simulink model "Forward_and_inverse_Both"  (R2024b)
settings: Solver=VariableStepAuto  StartTime=0.0  StopTime=7  MaxStep=0.005  RelTol=1e-3
model workspace: external: MATLAB File D:\OneDrive - itc.edu.kh\V4_robot_arm\Import_arm6\Test_Assembly_DataFile.m (data not in the file)
values from neighbouring files (symbols this model uses):
  Reach_max = max(REACH_MAX)    [Workspace_sample.m]
  Reach_min = max(REACH_MIN)    [Workspace_sample.m]
undefined symbols (not defined in the file or in its folder): DiscIntNeverNeededParam, initialPose, maxAngularAcc, maxAngularVel, maxLinearAcc, maxLinearVel, poseTol, smiData, Ts, wps1, X, Y, Z
libraries: sm_lib x140, nesl_utility x52, stmnucleolib x12, simulink x4, vrlib x2, vexcommonlib x2, robotcorelib x2
(part 5 of 6)

== system Forward_and_inverse_Both/Simscape Robot2/Link4_v2_1_RIGID1 ==
  ReferenceFrame : sm_lib/Frames and Transforms/Reference Frame
  Solid : sm_lib/Body Elements/File Solid  ExtGeomFileName=D:\Test_hardware\simscape\Solidworks FIle\Link4_v2_Default_sldprt.STEP  UnitType=FromFile  ExtGeomFileUnits=m  StepReaderType=HEX  ExportConvexHullGeometry=off  InertiaType=Custom  BasedOnType=DensityFromFile  Density=1000  DensityUnits=kg/m^3  Mass=smiData.Solid(7).mass  MassUnits=kg  CenterOfMass=smiData.Solid(7).CoM  CenterOfMassUnits=mm  MomentsOfInertia=smiData.Solid(7).MoI  MomentsOfInertiaUnits=kg*mm^2  ProductsOfInertia=smiData.Solid(7).PoI  ProductsOfInertiaUnits=kg*mm^2  GraphicType=FromGeometry  MarkerShape=Sphere  MarkerSize=10  GraphicVisPropType=SimpleVisualProperties  GraphicDiffuseColor=[0.0 1.0 1.0]  GraphicOpacity=smiData.Solid(7).opacity  GraphicSpecularColor=[0.1 0.1 0.1 1.0]  GraphicAmbientColor=[0.15 0.15 0.15 1.0]  GraphicEmissiveColor=[0.5 0.5 0.5 1.0]  GraphicShininess=75  DoExposeReferenceFrame=on  SerializedFrames=<Frames/>
  Transform : sm_lib/Frames and Transforms/Rigid Transform  RotationMethod=ArbitraryAxis  FollAlignAxisA=+X  BaseAlignAxisA=+Y  FollAlignAxisB=+Y  BaseAlignAxisB=+Z  RotationStandardAxis=+Z  RotationAngle=smiData.RigidTransform(2).angle  RotationAngleUnits=rad  RotationArbitraryAxis=smiData.RigidTransform(2).axis  RotationSequenceAxes=FollowerAxes  RotationSequence=XYX  RotationSequenceAngles=[0 0 0]  RotationSequenceAnglesUnits=deg  RotationMatrix=[1 0 0; 0 1 0; 0 0 1]  Quaternion=[1 0 0 0]  TranslationMethod=Cartesian  TranslationCartesianOffset=smiData.RigidTransform(2).translation  TranslationCartesianOffsetUnits=mm  TranslationStandardAxis=+Z  TranslationStandardOffset=0  TranslationStandardOffsetUnits=mm  TranslationROffset=0  TranslationROffsetUnits=m  TranslationThetaOffset=0  TranslationThetaOffsetUnits=deg  TranslationZOffset=0  TranslationZOffsetUnits=m
  Transform1 : sm_lib/Frames and Transforms/Rigid Transform  RotationMethod=ArbitraryAxis  FollAlignAxisA=+X  BaseAlignAxisA=+Y  FollAlignAxisB=+Y  BaseAlignAxisB=+Z  RotationStandardAxis=+Z  RotationAngle=smiData.RigidTransform(3).angle  RotationAngleUnits=rad  RotationArbitraryAxis=smiData.RigidTransform(3).axis  RotationSequenceAxes=FollowerAxes  RotationSequence=XYX  RotationSequenceAngles=[0 0 0]  RotationSequenceAnglesUnits=deg  RotationMatrix=[1 0 0; 0 1 0; 0 0 1]  Quaternion=[1 0 0 0]  TranslationMethod=Cartesian  TranslationCartesianOffset=smiData.RigidTransform(3).translation  TranslationCartesianOffsetUnits=mm  TranslationStandardAxis=+Z  TranslationStandardOffset=0  TranslationStandardOffsetUnits=mm  TranslationROffset=0  TranslationROffsetUnits=m  TranslationThetaOffset=0  TranslationThetaOffsetUnits=deg  TranslationZOffset=0  TranslationZOffsetUnits=m
  F : PMIOPort  Side=Left
  F1 : PMIOPort  Port=2  Side=Right
  connections:
  ReferenceFrame/RConn1 -- Transform/LConn1 -- Transform1/LConn1 -- Solid/RConn1
  Transform/RConn1 -- F/RConn1
  Transform1/RConn1 -- F1/RConn1

== system Forward_and_inverse_Both/Simscape Robot2/Link5_v2_1_RIGID1 ==
  ReferenceFrame : sm_lib/Frames and Transforms/Reference Frame
  Solid : sm_lib/Body Elements/File Solid  ExtGeomFileName=D:\Test_hardware\simscape\Solidworks FIle\Link5_v2_Default_sldprt.STEP  UnitType=FromFile  ExtGeomFileUnits=m  StepReaderType=HEX  ExportConvexHullGeometry=off  InertiaType=Custom  BasedOnType=DensityFromFile  Density=1000  DensityUnits=kg/m^3  Mass=smiData.Solid(1).mass  MassUnits=kg  CenterOfMass=smiData.Solid(1).CoM  CenterOfMassUnits=mm  MomentsOfInertia=smiData.Solid(1).MoI  MomentsOfInertiaUnits=kg*mm^2  ProductsOfInertia=smiData.Solid(1).PoI  ProductsOfInertiaUnits=kg*mm^2  GraphicType=FromGeometry  MarkerShape=Sphere  MarkerSize=10  GraphicVisPropType=SimpleVisualProperties  GraphicDiffuseColor=[0.2 1.0 1.0]  GraphicOpacity=smiData.Solid(1).opacity  GraphicSpecularColor=[0.5 0.5 0.5 1.0]  GraphicAmbientColor=[0.15 0.15 0.15 1.0]  GraphicEmissiveColor=[0.0 0.0 0.0 1.0]  GraphicShininess=75  DoExposeReferenceFrame=on  SerializedFrames=<Frames/>
  Transform : sm_lib/Frames and Transforms/Rigid Transform  RotationMethod=ArbitraryAxis  FollAlignAxisA=+X  BaseAlignAxisA=+Y  FollAlignAxisB=+Y  BaseAlignAxisB=+Z  RotationStandardAxis=+Z  RotationAngle=smiData.RigidTransform(4).angle  RotationAngleUnits=rad  RotationArbitraryAxis=smiData.RigidTransform(4).axis  RotationSequenceAxes=FollowerAxes  RotationSequence=XYX  RotationSequenceAngles=[0 0 0]  RotationSequenceAnglesUnits=deg  RotationMatrix=[1 0 0; 0 1 0; 0 0 1]  Quaternion=[1 0 0 0]  TranslationMethod=Cartesian  TranslationCartesianOffset=smiData.RigidTransform(4).translation  TranslationCartesianOffsetUnits=mm  TranslationStandardAxis=+Z  TranslationStandardOffset=0  TranslationStandardOffsetUnits=mm  TranslationROffset=0  TranslationROffsetUnits=m  TranslationThetaOffset=0  TranslationThetaOffsetUnits=deg  TranslationZOffset=0  TranslationZOffsetUnits=m
  Transform1 : sm_lib/Frames and Transforms/Rigid Transform  RotationMethod=ArbitraryAxis  FollAlignAxisA=+X  BaseAlignAxisA=+Y  FollAlignAxisB=+Y  BaseAlignAxisB=+Z  RotationStandardAxis=+Z  RotationAngle=smiData.RigidTransform(9).angle  RotationAngleUnits=rad  RotationArbitraryAxis=smiData.RigidTransform(9).axis  RotationSequenceAxes=FollowerAxes  RotationSequence=XYX  RotationSequenceAngles=[0 0 0]  RotationSequenceAnglesUnits=deg  RotationMatrix=[1 0 0; 0 1 0; 0 0 1]  Quaternion=[1 0 0 0]  TranslationMethod=Cartesian  TranslationCartesianOffset=smiData.RigidTransform(9).translation  TranslationCartesianOffsetUnits=mm  TranslationStandardAxis=+Z  TranslationStandardOffset=0  TranslationStandardOffsetUnits=mm  TranslationROffset=0  TranslationROffsetUnits=m  TranslationThetaOffset=0  TranslationThetaOffsetUnits=deg  TranslationZOffset=0  TranslationZOffsetUnits=m
  F : PMIOPort  Side=Left
  F1 : PMIOPort  Port=2  Side=Right
  connections:
  ReferenceFrame/RConn1 -- Transform/LConn1 -- Transform1/LConn1 -- Solid/RConn1
  Transform/RConn1 -- F/RConn1
  Transform1/RConn1 -- F1/RConn1

== system Forward_and_inverse_Both/Subsystem/Joint 1 R1 = counter-clockwise L1 = clockwise ==
  L1 : Inport
  R1 : Inport  Port=2
  delta : Inport  Port=3
  pos_prev : Inport  Port=4
  MATLAB Function1 : MATLAB Function  TreatAsAtomicUnit=on
  Position limiter : MATLAB Function  TreatAsAtomicUnit=on
  Joint_1 : Outport
  wires:
  R1/1 -> MATLAB Function1/2(buttonR)
  Position limiter/1(y) -> Joint_1/1
  MATLAB Function1/1(pos) -> Position limiter/1(pos)
  L1/1 -> MATLAB Function1/1(buttonL)
  delta/1 -> Position limiter/2(delta), MATLAB Function1/4(delta)
  pos_prev/1 -> MATLAB Function1/3(pos_prev)

== system Forward_and_inverse_Both/Subsystem/Joint 6 L = counter-clockwise R = clockwise ==
  Dpad L : Inport
  Dpad R : Inport  Port=2
  delta : Inport  Port=3
  pos_prev : Inport  Port=4
  MATLAB Function1 : MATLAB Function  TreatAsAtomicUnit=on
  Position limiter : MATLAB Function  TreatAsAtomicUnit=on
  Joint_6 : Outport
  wires:
  delta/1 -> MATLAB Function1/4(delta), Position limiter/2(delta)
  Dpad L/1 -> MATLAB Function1/1(buttonL)
  MATLAB Function1/1(pos) -> Position limiter/1(pos)
  Position limiter/1(y) -> Joint_6/1
  Dpad R/1 -> MATLAB Function1/2(buttonR)
  pos_prev/1 -> MATLAB Function1/3(pos_prev)

== system Forward_and_inverse_Both/Subsystem20/Joint 1 R1 = counter-clockwise L1 = clockwise ==
  L1 : Inport
  R1 : Inport  Port=2
  delta : Inport  Port=3
  pos_prev : Inport  Port=4
  MATLAB Function1 : MATLAB Function  TreatAsAtomicUnit=on
  Position limiter : MATLAB Function  TreatAsAtomicUnit=on
  Joint_1 : Outport
  wires:
  R1/1 -> MATLAB Function1/2(buttonR)
  Position limiter/1(y) -> Joint_1/1
  MATLAB Function1/1(pos) -> Position limiter/1(pos)
  L1/1 -> MATLAB Function1/1(buttonL)
  delta/1 -> Position limiter/2(delta), MATLAB Function1/4(delta)
  pos_prev/1 -> MATLAB Function1/3(pos_prev)

== system Forward_and_inverse_Both/Subsystem20/Joint 6 L = counter-clockwise R = clockwise ==
  Dpad L : Inport
  Dpad R : Inport  Port=2
  delta : Inport  Port=3
  pos_prev : Inport  Port=4
  MATLAB Function1 : MATLAB Function  TreatAsAtomicUnit=on
  Position limiter : MATLAB Function  TreatAsAtomicUnit=on
  Joint_6 : Outport
  wires:
  delta/1 -> MATLAB Function1/4(delta), Position limiter/2(delta)
  Dpad L/1 -> MATLAB Function1/1(buttonL)
  MATLAB Function1/1(pos) -> Position limiter/1(pos)
  Position limiter/1(y) -> Joint_6/1
  Dpad R/1 -> MATLAB Function1/2(buttonR)
  pos_prev/1 -> MATLAB Function1/3(pos_prev)

== matlab function Forward_and_inverse_Both/Forward_Kinematic_Good4 ==
  data: Px output; Py output; Pz output; th1 input; th2 input; th3 input; th4 input; th5 input; th6 input
function [Px,Py,Pz] = forward_kinematics(th1, th2, th3, th4, th5, th6)
%All length in mm
l1=276;
l2=306;
a=79.75;
l3=160;
l4=227;
l5=70;
l6=38;
    % Compute DH transformation matrices
    A0 = dh_matrix(0    , 0     ,l1 , th1);   
    A1 = dh_matrix(0    ,-pi/2  ,0  , th2-pi/2);
    A2 = dh_matrix(l2   ,0      ,0  ,th3);
%     A3p= dh_matrix(a   ,0      ,0, 0);
    A3 = dh_matrix(a    ,-pi/2  ,0  ,th4);
    A4 = dh_matrix(0    ,0      ,l3+l4 ,0);
    A4p= dh_matrix(0   ,pi/2   ,0  ,th5);
    A5 = dh_matrix(0    ,-pi/2  , 0 ,th6);
    A6 = dh_matrix(0    ,0      ,l5+l6 ,0);
    
    % Total forward matrix H
    A0_6 = ( A0*A1 * A2 * A3 * A4 * A4p * A5 * A6) ;
    Px=A0_6(1,4);
    Py=A0_6(2,4);
    Pz=A0_6(3,4);

end
function A = dh_matrix(a , alpha ,d ,theta)
    A = [cos(theta)            , -sin(theta),           0       ,   a;
         cos(alpha)*sin(theta), cos(theta)*cos(alpha), -sin(alpha), -d*sin(alpha);
         sin(alpha)*sin(theta), sin(alpha)*cos(theta), cos(alpha), d*cos(alpha);
         0, 0, 0, 1];
end

== matlab function Forward_and_inverse_Both/Forward_Kinematic ==
  data: th1 input; th2 input; th3 input; th4 input; th5 input; th6 input; A0_6 output
function A0_6  = forward_kinematics(th1, th2, th3, th4, th5, th6)
% 
% %     Define DH parameters
%     l1 = 276/1000;  % Length of link 1
%     l2 = 305.94661/1000 ;
%     l3 = 154.46177/1000;
%     l4 =228.74688/1000;% Length of link 2
%     l5 = 68.15773/1000;
%     l6=41.47212/1000 ;   % Length of link 6
%     a= 82.4965/1000;
%old length all in mm
 l1=276;
l2=306;
a=79.75;
l3=160;
l4=227;
l5=70;
l6=38;
    % Compute DH transformation matrices
    A0 = dh_matrix(0    , 0     ,l1 , th1);   
    A1 = dh_matrix(0    ,-pi/2  ,0  , th2-pi/2);
    A2 = dh_matrix(l2   ,0      ,0  ,th3);
%     A3p= dh_matrix(a   ,0      ,0, 0);
    A3 = dh_matrix(a    ,-pi/2  ,0  ,th4);
    A4 = dh_matrix(0    ,0      ,l3+l4 ,0);
    A4p= dh_matrix(0   ,pi/2   ,0  ,th5);
    A5 = dh_matrix(0    ,-pi/2  , 0 ,th6);
    A6 = dh_matrix(0    ,0      ,l5+l6 ,0);
    
    % Total forward matrix H
    A0_6 = ( A0*A1 * A2 * A3 * A4 * A4p * A5 * A6) ;

    R06 =(A0_6(1:3,1:3));
    A03=A0*A1*A2;
    R03=(A03(1:3,1:3));
    A3_6= A3*A4*A4p*A5*A6;
    R36=(A3_6(1:3,1:3));

    Px=A0_6(1,4);
    Py=A0_6(2,4);
    Pz=A0_6(3,4);

end
function A = dh_matrix(a , alpha ,d ,theta)
    A = [cos(theta)            , -sin(theta),           0       ,   a;
         cos(alpha)*sin(theta), cos(theta)*cos(alpha), -sin(alpha), -d*sin(alpha);
         sin(alpha)*sin(theta), sin(alpha)*cos(theta), cos(alpha), d*cos(alpha);
         0, 0, 0, 1];
end

== matlab function Forward_and_inverse_Both/Forward_Kinematic_Good3 ==
  data: Px output; Py output; Pz output; th1 input; th2 input; th3 input; th4 input; th5 input; th6 input
function [Px,Py,Pz] = forward_kinematics(th1, th2, th3, th4, th5, th6)
% 
% %     Define DH parameters
%     l1 = 276/1000;  % Length of link 1
%     l2 = 305.94661/1000 ;
%     l3 = 154.46177/1000;
%     l4 =228.74688/1000;% Length of link 2
%     l5 = 68.15773/1000;
%     l6=41.47212/1000 ;   % Length of link 6
%     a= 82.4965/1000;
%old length all in mm
l1=276;
l2=306;
a=79.75;
l3=160;
l4=227;
l5=70;
l6=38;
    % Compute DH transformation matrices
    A0 = dh_matrix(0    , 0     ,l1 , th1);   
    A1 = dh_matrix(0    ,-pi/2  ,0  , th2-pi/2);
    A2 = dh_matrix(l2   ,0      ,0  ,th3);
%     A3p= dh_matrix(a   ,0      ,0, 0);
    A3 = dh_matrix(a    ,-pi/2  ,0  ,th4);
    A4 = dh_matrix(0    ,0      ,l3+l4 ,0);
    A4p= dh_matrix(0   ,pi/2   ,0  ,th5);
    A5 = dh_matrix(0    ,-pi/2  , 0 ,th6);
    A6 = dh_matrix(0    ,0      ,l5+l6 ,0);
    
    % Total forward matrix H
    A0_6 = ( A0*A1 * A2 * A3 * A4 * A4p * A5 * A6) ;
%     R06 =(A0_6(1:3,1:3));
%     A03=A0*A1*A2;
%     R03=(A03(1:3,1:3));
%     A3_6= A3p*A3*A4*A4p*A5*A6;
%     R36=(A3_6(1:3,1:3));
 
    Px=A0_6(1,4);
    Py=A0_6(2,4);
    Pz=A0_6(3,4);

end
function A = dh_matrix(a , alpha ,d ,theta)
    A = [cos(theta)            , -sin(theta),           0       ,   a;
         cos(alpha)*sin(theta), cos(theta)*cos(alpha), -sin(alpha), -d*sin(alpha);
         sin(alpha)*sin(theta), sin(alpha)*cos(theta), cos(alpha), d*cos(alpha);
         0, 0, 0, 1];
end

== matlab function Forward_and_inverse_Both/Rotation Matrix ==
  data: roll input; R06 output
function R06 = fcn(roll)

yaw   = pi;
pitch = -pi/2;

Rx   = [1    0         0
        0   cos(roll)  -sin(roll)
        0   sin(roll)   cos(roll)];
Ry   = [cos(pitch)   0   sin(pitch)
           0         1      0
        -sin(pitch)  0   cos(pitch)];
Rz   = [cos(yaw)  -sin(yaw)   0
        sin(yaw)   cos(yaw)   0
          0           0       1];

R06  = Rz*Ry*Rx;

== matlab function Forward_and_inverse_Both/Subsystem15/Define Relative angle1 ==
  settings: updateMethod=DISCRETE
  data: initialPose input; reset_angle input; rawangle input; angle output; status input
function angle = fcn(initialPose, reset_angle, rawangle, status)

% continuousangle is absolute angle
% angle is relative angle

persistent prevPsi2pi jump rawangle_0 set_angle
if isempty(prevPsi2pi)
    prevPsi2pi = 0; jump = 0; rawangle_0 = rawangle; set_angle = 0;
end

if abs(rawangle-prevPsi2pi) >  pi
    if rawangle > 0
        jump = jump - 1;
    else
        jump = jump + 1;
    end
end
prevPsi2pi = rawangle;

continuousangle = rawangle + jump*2*pi; % continuous value

if (status && ~set_angle), rawangle_0 = continuousangle; set_angle  = 1; end

if reset_angle, rawangle_0 = continuousangle; end

angle = continuousangle - rawangle_0 + initialPose;

== matlab function Forward_and_inverse_Both/Inverse Kinematic2 ==
  settings: updateMethod=DISCRETE
  data: Px input; q1 output; Py input; Pz input; q2 output; q3 output; q4 output; q5 output; q6 output; R06 input
function [q1, q2, q3, q4, q5, q6] = inverseKinematics(Px, Py, Pz, R06)
    % Define actual geometry parameters (in mm)
    l1=276;
    l2=306;
    a=79.75;
    l3=160;
    l4=227;
    l5=70;
    l6=38;
    % Wrist position calculation
    O6=[Px,Py,Pz]';
    d6=l5+l6;
    OW = O6 - R06*[0;0;d6];
    % Compute wrist position (compensating for the end-effector offset)
    Pwx=OW(1);
    Pwy=OW(2);
    Pwz=OW(3);
    % Compute q1 directly from the wrist position
    q1 = atan2(Pwy, Pwx);
    r = sqrt(Pwx^2 + Pwy^2);
    h= Pwz-l1;
    % Intermediate calculations for q2 and q3
    s = sqrt(h^2 + r^2);
    alp = atan(h/r );
    w3 = l3 + l4;
    k3 = sqrt(a^2 + w3^2);
    beta = acos((l2^2 + s^2 - k3^2) / (2 * l2 * s));
    gamma = acos(( l2^2+k3^2-s^2) / (2 * l2 * k3));
    Phi = atan(w3/a);
    % Target angles for q2 and q3
    q2 = (-alp -beta+pi/2);
    q3 = (pi-gamma - Phi);

    % Compute R0_3 from q1, q2, q3
    R03 = [cos(q1)*cos(q2 + q3), -cos(q1)*sin(q2 + q3), -sin(q1);
           sin(q1)*cos(q2 + q3), -sin(q1)*sin(q2 + q3),  cos(q1);
           -sin(q2 + q3)       , -cos(q2 + q3)        , 0 ];
    R03t=transpose(R03);

    % Compute R3_6 from the known R0_3 and R0_6
    R3_6 = R03t* R06;

    % Extract elements from R3_6 for calculating q4, q5, q6
    s5c4 = -R3_6(1, 3);
    c5   = R3_6(2, 3);
    s5s4 = R3_6(3, 3);
    s5c6 = R3_6(2, 1);
    s5s6 = -R3_6(2, 2);

    % Joint angle q5

      q5p = atan2(-sqrt(1-c5^2),c5);
 % Joint angles q4 and q6
      q5=q5p;
        q4 = atan2(-s5s4, -s5c4);
        q6 = atan2(-s5s6, -s5c6);

end

== matlab function Forward_and_inverse_Both/Set Joint position to where it were left off/limit J2 & J3 so that it won't collide with itself/Joint2 ==
  data: pos input; delta input; posfinal output; pos_prev input
function posfinal = fcn(pos,delta,pos_prev)

if pos > 0        %%In case of clockwise rotation
    posc = pos_prev + abs(delta);
elseif pos < 0    %%In case of counter clockwise rotation
    posc = pos_prev - abs(delta);
else               %%Stay still if there's no input
    posc = pos_prev;
end

if posc <= 1 && posc >= -1.2 %%The joint only update its position if it stays within this range
    posfinal = posc;
else
    posfinal = pos_prev;
end

== matlab function Forward_and_inverse_Both/Forward_Kinematic_Good2 ==
  data: th1 input; th2 input; th3 input; th4 input; th5 input; th6 input; A06 output; R06 output; R03 output; R36 output
function [A06, R06,R03,R36] = forward_kinematics(th1, th2, th3, th4, th5, th6)

    % Define DH parameters
   l1 = 276/1000;  % Length of link 1
    l2 = 305.94661/1000 ;
    l4 = (154.46177+228.74688)/1000;% Length of link 2
    l6 = (68.15773+41.47212)/1000 ;   % Length of link 6
    a= 82.4965/1000;
    
    % Compute DH transformation matrices
    A0 = dh_matrix(0    , 0     ,l1 , th1);   
    A1 = dh_matrix(0    ,-pi/2  ,0  , th2 );
    A2 = dh_matrix(l2   ,0      ,0  ,th3);
    A3 = dh_matrix(a    ,-pi/2  ,0  ,th4);
    A4 = dh_matrix(0    ,0      ,l4 ,0);
    A4p= dh_matrix(0   ,pi/2   ,0  ,th5);
    A5 = dh_matrix(0    ,-pi/2  , 0 ,th6);
    A6 = dh_matrix(0    ,0      ,l6 ,0);
    
    % Total forward matrix H
    A06 = A0*A1 * A2 * A3 * A4 * A4p * A5 * A6 ;
    R06 =round(A06(1:3,1:3));
    A03=A0*A1 * A2 * A3 * A4 * A4p * A5;
    R03=round(A03(1:3,1:3));
    A36= A03.'*A06;
    R36=round(A36(1:3,1:3));



   
    Px=A06(1,4);
    Py=A06(2,4);
    Pz=A06(3,4);

end
function A = dh_matrix(a , alpha ,d ,theta)
    A = [cos(theta)            , -sin(theta),           0       ,   a;
         cos(alpha)*sin(theta), cos(theta)*cos(alpha), -sin(alpha), -d*sin(alpha);
         sin(alpha)*sin(theta), sin(alpha)*cos(theta), cos(alpha), d*cos(alpha);
         0, 0, 0, 1];
end

== matlab function Forward_and_inverse_Both/Subsystem/Joint 1 R1 = counter-clockwise L1 = clockwise/MATLAB Function1 ==
  data: buttonL input; buttonR input; pos output; pos_prev input; delta input
function pos = fcn(buttonL,buttonR, pos_prev,delta)

    if buttonR == 1 && buttonL == 0

        pos = pos_prev + delta;
    elseif buttonR == 0 && buttonL == 1
    
        pos = pos_prev - delta;
    else
        pos = pos_prev;
    end
end

== matlab function Forward_and_inverse_Both/Subsystem/Joint 1 R1 = counter-clockwise L1 = clockwise/Position limiter ==
  data: pos input; delta input; y output
function y = fcn(pos,delta)

if pos <= -1.3
    pos = pos + delta; %pos = pos_prev
elseif pos >= 1.3
    pos = pos - delta;
end

y = pos;

== matlab function Forward_and_inverse_Both/Set Delta for the joint movement more Delta, faster the movement/ speed setting ==
  data: O input; Tri input; y output; delta input
function y = fcn(O,Tri,delta)

    if O == 1 && Tri ==0 && delta <= 0.1
        delta = delta + 0.025;
    elseif Tri == 1 && O == 0 && delta >= 0.025
        delta = delta - 0.025;
    else
    end
    y = delta;
end

== matlab function Forward_and_inverse_Both/Subsystem1/MATLAB Function ==
  data: goal input; Msg output; speedMode input; stop input; reset input; voltageMode input
function Msg = fcn(goal, speedMode, stop, reset, voltageMode)
    Msg = uint8(zeros(8,1));

    Msg(1) = speedMode + stop * 2 + reset * 4 + voltageMode * 8;

    Msg(3:6) = typecast(single(goal), 'uint8');
end

== matlab function Forward_and_inverse_Both/Subsystem2/MATLAB Function ==
  data: goal input; Msg output; speedMode input; stop input; reset input; voltageMode input
function Msg = fcn(goal, speedMode, stop, reset, voltageMode)
    Msg = uint8(zeros(8,1));

    Msg(1) = speedMode + stop * 2 + reset * 4 + voltageMode * 8;

    Msg(3:6) = typecast(single(goal), 'uint8');
end

== matlab function Forward_and_inverse_Both/Subsystem3/MATLAB Function ==
  data: goal input; Msg output; speedMode input; stop input; reset input; voltageMode input
function Msg = fcn(goal, speedMode, stop, reset, voltageMode)
    Msg = uint8(zeros(8,1));

    Msg(1) = speedMode + stop * 2 + reset * 4 + voltageMode * 8;

    Msg(3:6) = typecast(single(goal), 'uint8');
end

== matlab function Forward_and_inverse_Both/Subsystem5/MATLAB Function ==
  data: goal input; Msg output; speedMode input; stop input; reset input; voltageMode input
function Msg = fcn(goal, speedMode, stop, reset, voltageMode)
    Msg = uint8(zeros(8,1));

    Msg(1) = speedMode + stop * 2 + reset * 4 + voltageMode * 8;

    Msg(3:6) = typecast(single(goal), 'uint8');
end

== matlab function Forward_and_inverse_Both/Subsystem6/MATLAB Function ==
  data: goal input; Msg output; speedMode input; stop input; reset input; voltageMode input
function Msg = fcn(goal, speedMode, stop, reset, voltageMode)
    Msg = uint8(zeros(8,1));

    Msg(1) = speedMode + stop * 2 + reset * 4 + voltageMode * 8;

    Msg(3:6) = typecast(single(goal), 'uint8');
end

== matlab function Forward_and_inverse_Both/Subsystem10/MATLAB Function ==
  data: data input; position output; speed output
function [position, speed] = fcn(data)
    %#codegen
    position = zeros(1, 1, 'single');
    speed = zeros(1, 1, 'single');

    if numel(data) >= 8
        position = typecast(data(1:4), 'single');
        speed = typecast(data(5:8), 'single');
    end
end

== matlab function Forward_and_inverse_Both/Subsystem11/MATLAB Function ==
  data: data input; position output; speed output
function [position, speed] = fcn(data)
    %#codegen
    position = zeros(1, 1, 'single');
    speed = zeros(1, 1, 'single');

    if numel(data) >= 8
        position = typecast(data(1:4), 'single');
        speed = typecast(data(5:8), 'single');
    end
end

== matlab function Forward_and_inverse_Both/Subsystem4/MATLAB Function ==
  data: goal input; Msg output; speedMode input; stop input; reset input; voltageMode input
function Msg = fcn(goal, speedMode, stop, reset, voltageMode)
    Msg = uint8(zeros(8,1));

    Msg(1) = speedMode + stop * 2 + reset * 4 + voltageMode * 8;

    Msg(3:6) = typecast(single(goal), 'uint8');
end

== matlab function Forward_and_inverse_Both/Subsystem12/MATLAB Function ==
  data: data input; position output; speed output
function [position, speed] = fcn(data)
    %#codegen
    position = zeros(1, 1, 'single');
    speed = zeros(1, 1, 'single');

    if numel(data) >= 8
        position = typecast(data(1:4), 'single');
        speed = typecast(data(5:8), 'single');
    end
end

== matlab function Forward_and_inverse_Both/Subsystem7/MATLAB Function ==
  data: data input; position output; speed output
function [position, speed] = fcn(data)
    %#codegen
    position = zeros(1, 1, 'single');
    speed = zeros(1, 1, 'single');

    if numel(data) >= 8
        position = typecast(data(1:4), 'single');
        speed = typecast(data(5:8), 'single');
    end
end

== matlab function Forward_and_inverse_Both/Subsystem8/MATLAB Function ==
  data: data input; position output; speed output
function [position, speed] = fcn(data)
    %#codegen
    position = zeros(1, 1, 'single');
    speed = zeros(1, 1, 'single');

    if numel(data) >= 8
        position = typecast(data(1:4), 'single');
        speed = typecast(data(5:8), 'single');
    end
end

== matlab function Forward_and_inverse_Both/Subsystem9/MATLAB Function ==
  data: data input; position output; speed output
function [position, speed] = fcn(data)
    %#codegen
    position = zeros(1, 1, 'single');
    speed = zeros(1, 1, 'single');

    if numel(data) >= 8
        position = typecast(data(1:4), 'single');
        speed = typecast(data(5:8), 'single');
    end
end

== matlab function Forward_and_inverse_Both/Subsystem/Joint 6 L = counter-clockwise R = clockwise/MATLAB Function1 ==
  data: buttonL input; buttonR input; pos output; pos_prev input; delta input
function pos = fcn(buttonL,buttonR, pos_prev,delta)

    if buttonR == 1 && buttonL == 0

        pos = pos_prev - delta*1.25;
    elseif buttonR == 0 && buttonL == 1
    
        pos = pos_prev + delta*1.25;
    else
        pos = pos_prev;
    end
end

== matlab function Forward_and_inverse_Both/Flip the state of a button/MATLAB Function1 ==
  data: y output; X input; delta input; n input; error output
function [y , error] = fcn(X,delta,n)

    if X == 1 && n <= 2
        delta = 0;
        n = n + 1;
    elseif X == 1 && n > 2
        delta = 0;
        n = 0;
    elseif X == 0
        n = 0;
        delta = 1;
    end
    y = delta;
    error = n;
end

== matlab function Forward_and_inverse_Both/Set Joint position to where it were left off/limit J2 & J3 so that it won't collide with itself/Joint1 ==
  data: pos input; posfinal output; pos_prev input; delta input
function posfinal = fcn(pos,pos_prev,delta)

if pos > 0        %%In case of clockwise rotation
    posc = pos_prev + abs(delta);
elseif pos < 0    %%In case of counter clockwise rotation
    posc = pos_prev - abs(delta);
else               %%Stay still if there's no input
    posc = pos_prev;
end

if posc <= 1 && posc >= -1.2 %%The joint only update its position if it stays within this range
    posfinal = posc;
else
    posfinal = pos_prev;
end

== matlab function Forward_and_inverse_Both/Set Joint position to where it were left off/limit J2 & J3 so that it won't collide with itself/MATLAB Function1 ==
  data: delta input; n input; y output; pos input; pos_prev input
function y = fcn(delta,n,pos,pos_prev)
if n == 0 && pos > 0
    pos = max(0,pos_prev - abs(delta));
elseif n == 0 && pos < 0
    pos = min(0,pos_prev + abs(delta));
end
y = pos;

== matlab function Forward_and_inverse_Both/Subsystem16/Define Relative angle1 ==
  settings: updateMethod=DISCRETE
  data: initialPose input; reset_angle input; rawangle input; angle output; status input
function angle = fcn(initialPose, reset_angle, rawangle, status)

% continuousangle is absolute angle
% angle is relative angle

persistent prevPsi2pi jump rawangle_0 set_angle
if isempty(prevPsi2pi)
    prevPsi2pi = 0; jump = 0; rawangle_0 = rawangle; set_angle = 0;
end

if abs(rawangle-prevPsi2pi) >  pi
    if rawangle > 0
        jump = jump - 1;
    else
        jump = jump + 1;
    end
end
prevPsi2pi = rawangle;

continuousangle = rawangle + jump*2*pi; % continuous value

if (status && ~set_angle), rawangle_0 = continuousangle; set_angle  = 1; end

if reset_angle, rawangle_0 = continuousangle; end

angle = continuousangle - rawangle_0 + initialPose;

== matlab function Forward_and_inverse_Both/Set Joint position to where it were left off/Joint3 ==
  data: pos input; posfinal output; pos_prev input; delta input
function posfinal = fcn(pos,pos_prev,delta)

if pos > 0        %%In case of clockwise rotation
    posc = pos_prev + abs(delta);
elseif pos < 0    %%In case of counter clockwise rotation
    posc = pos_prev - abs(delta);
else               %%Stay still if there's no input
    posc = pos_prev;
end

if posc <= 1 && posc >= -1.2 %%The joint only update its position if it stays within this range
    posfinal = posc;
else
    posfinal = pos_prev;
end

== matlab function Forward_and_inverse_Both/Subsystem/Joint 6 L = counter-clockwise R = clockwise/Position limiter ==
  data: pos input; delta input; y output
function y = fcn(pos,delta)

if pos <= -1.3
    pos = pos + delta; %pos = pos_prev
elseif pos >= 1.3
    pos = pos - delta;
end

y = pos;

== matlab function Forward_and_inverse_Both/Set Joint position to where it were left off/limit J2 & J3 so that it won't collide with itself/MATLAB Function ==
  data: delta input; n input; y output; pos input; pos_prev input
function y = fcn(delta,n,pos,pos_prev)
if n == 0 && pos > 0
    pos = max(0,pos_prev - abs(delta));
elseif n == 0 && pos < 0
    pos = min(0,pos_prev + abs(delta));
end
y = pos;

== matlab function Forward_and_inverse_Both/Set Joint position to where it were left off/MATLAB Function2 ==
  data: delta input; n input; y output; pos input; pos_prev input
function y = fcn(delta,n,pos,pos_prev)
if n == 0 && pos > 0
    pos = max(0,pos_prev - abs(delta));
elseif n == 0 && pos < 0
    pos = min(0,pos_prev + abs(delta));
end
y = pos;

== matlab function Forward_and_inverse_Both/Inverse Kinematic1 ==
  settings: updateMethod=DISCRETE
  data: Px input; q1 output; Py input; Pz input; q2 output; q3 output; q4 output; q5 output; q6 output; R06 input
function [q1, q2, q3, q4, q5, q6] = inverseKinematics(Px, Py, Pz, R06)
    % Define actual geometry parameters (in meters)
%     l1 = 276;        % Length of link 1
%     l2 = 305.94661;  % Length of link 2
%     l3 = 154.46177;  % Length of link 3
%     l4 = 228.74688;  % Length of link 4
%     l5 = 68.15773;   % Length of link 5 (offset)
%     l6 = 41.47212;   % Length of link 6 (end-effector)
%     a  = 82.4965;    % Offset a
%%Old length 
l1=276;
l2=306;
a=79.75;
l3=160;
l4=227;
l5=70;
l6=38;

%     R06=[0    0   1
%          0   -1   0
%          1    0   0];
    % Wrist position calculation
    O6=[Px,Py,Pz]';
    d6=l5+l6;
    OW = O6 - R06*[0;0;d6];
%     r13 = R06(1, 3);
%     r23 = R06(2, 3);
%     r33 = R06(3, 3);

    % Compute wrist position (compensating for the end-effector offset)
%     Pwx = Px - (l5 + l6) * r13;
%     Pwy = Py - (l5 + l6) * r23;
%     Pwz = Pz - (l5 + l6) * r33;
Pwx=OW(1); Pwy=OW(2);Pwz=OW(3);

    % Compute q1 directly from the wrist position
    q1 = atan2(Pwy, Pwx);

    % Convert wrist position to cylindrical coordinates
    r = sqrt(Pwx^2 + Pwy^2);
    %new code 
    h= Pwz-l1;
    % my code: h = Pwz - l1;

    % Intermediate calculations for q2 and q3
    s = sqrt(h^2 + r^2);
    alp = atan(h/r );
    w3 = l3 + l4;
    k3 = sqrt(a^2 + w3^2);
    %phi2
    beta = acos((l2^2 + s^2 - k3^2) / (2 * l2 * s));
   %gamma or phi3
    gamma = acos(( l2^2+k3^2-s^2) / (2 * l2 * k3));
    Phi = atan(w3/a);
    

    % Target angles for q2 and q3
    q2 = (-alp -beta+pi/2);
    q3 = (pi-gamma - Phi);
%     q3= -gamma-pi/2;

    % Compute R0_3 from q1, q2, q3
    R03 = [cos(q1)*cos(q2 + q3), -cos(q1)*sin(q2 + q3), -sin(q1);
           sin(q1)*cos(q2 + q3), -sin(q1)*sin(q2 + q3),  cos(q1);
           -sin(q2 + q3)       , -cos(q2 + q3)        , 0 ];
    R03t=transpose(R03);

    % Compute R3_6 from the known R0_3 and R0_6
    R3_6 = R03t* R06;

    % Extract elements from R3_6 for calculating q4, q5, q6
    s5c4 = -R3_6(1, 3);
    c5   = R3_6(2, 3);
    s5s4 = R3_6(3, 3);
    s5c6 = R3_6(2, 1);
    s5s6 = -R3_6(2, 2);

    % Joint angle q5
%     q5m = atan2(-sqrt(1 - c5^2), c5);
      q5p = atan2(-sqrt(1-c5^2),c5);
% q5p=asin(c5);
% 
%     % Joint angles q4 and q6 based on the sign of q5
%     if q5m > q5p
%        q5=q5m;
%     q5=q5p;
%        q4 = atan2(s5s4  , s5c4);
%        q6 = atan2(s5s6, s5c6);
%     else    
      q5=q5p;
        q4 = atan2(-s5s4, s5c4);
        q6 = atan2(-s5s6, -s5c6);
    
%     end
end

== stateflow chart Forward_and_inverse_Both/Waypoint Planner ==
  state Semi_auto
    en: wps = zeros(4,20); mode = auto ;
    du:
    state Delay1
    state Goto_up
      en:
      percentage = 10;
      moving(wps);
    (default) -> Goto_up : {move = 0; stage = 1;
        | col = width(wps1);
        | wps(:,2:col+1) = wps1;
        | wps(:,1) = genPose;}
    Goto_up -> Delay1 [order 1] : [semiAutoButton(1) &&...
        |  semiAutoButton(2)==1]
        | {move=0;
        | col = width(wps1);
        | wps(:,2:col+1) = wps1;
        | wps(:,1) = genPose;}
    Delay1 -> Goto_up : [after(3,sec)]
    Goto_up -> Goto_up [order 2] : [norm(targetPose - genPose)...
        | <poseTol && move<col]
  state Manual
    en:
    man = 0; auto = 1;
    departPose = genPose; stage = 0;
    targetPose  = genPose + [0;0;0;0];
    lastShotAng = 0; psi_inc = initialPose(4);
    maxVel        = [maxLinearVel , maxAngularVel];
    du:
  state moving(wayPoints) [function]
    (default) -> (junction 92) : {move = move+1;
        | departTime = t;
        | traject = wayPoints(:,2:end) - wayPoints(:,1:end-1);
        | departPose = genPose;
        | aheadPoint = traject(:,move);
        | psi_inc        = psi_inc + aheadPoint(4);
        | targetPose  = genPose+aheadPoint;
        | targetPose(4) = psi_inc - lastShotAng;
        | maxVel(1)   = percentage/100*maxLinearVel;
        | dist              = norm(aheadPoint(1:3));
        | deltaT          = dist/maxVel(1);
        | maxVel(2)   = min(maxAngularVel,...
        |                              abs(aheadPoint(4)/deltaT));}
  (default) -> Manual
  Manual -> Semi_auto : [semiAutoButton(1) &&...
      |  semiAutoButton(2)==1]
  data: wayPoints function_input; departTime output; departPose output; targetPose output; maxVel output; genPose input; maxLinearVel parameter; semiAutoButton input; poseTol parameter; mode output; dist local; auto local; man local; move local; aheadPoint local; deltaT local; maxAngularVel parameter; initialPose parameter; percentage local; lastShotAng local; stage local; psi_inc local; wps local; col local; wps1 parameter; traject local

== matlab function Forward_and_inverse_Both/Subsystem17/Define Relative angle ==
  settings: updateMethod=DISCRETE
  data: initialPose input; reset_angle input; rawangle input; angle output; status input
function angle = fcn(initialPose, reset_angle, rawangle, status)

% continuousangle is absolute angle
% angle is relative angle

persistent prevPsi2pi jump rawangle_0 set_angle
if isempty(prevPsi2pi)
    prevPsi2pi = 0; jump = 0; rawangle_0 = rawangle; set_angle = 0;
end

if abs(rawangle-prevPsi2pi) >  pi
    if rawangle > 0
        jump = jump - 1;
    else
        jump = jump + 1;
    end
end
if abs(rawangle-prevPsi2pi) >  pi/2 && abs(rawangle-prevPsi2pi) < pi
    if rawangle > 0
        jump = jump - 1/2;
    else
        jump = jump + 1/2;
    end
end

prevPsi2pi = rawangle;

continuousangle = rawangle + jump*2*pi; % continuous value

if (status && ~set_angle), rawangle_0 = continuousangle; set_angle  = 1; end

if reset_angle, rawangle_0 = continuousangle; end

angle = continuousangle - rawangle_0 + initialPose;

== matlab function Forward_and_inverse_Both/Waypoint Trajectory/3D Waypoint for Auto ==
  settings: updateMethod=DISCRETE
  data: genAcc output size=[4,1]; Ts output size=[1,1]; t input; departTime input; departPose input; targetPose input; maxVel input; maxAcc input
 function [genAcc,Ts] = fcn(t,departTime,departPose,targetPose,maxVel,maxAcc)
%#codegen

persistent  t1 prevVel
if isempty(t1)
    t1 = 0; prevVel = [0;0;0;0];
end

Ts = t-t1;
t1 = t;
maxLinearAcc    = abs(maxAcc(1));
maxAngularAcc   = abs(maxAcc(2));
maxLinearVel    = abs(maxVel(1));
maxAngularVel   = abs(maxVel(2));
if maxLinearAcc  == 0, maxLinearAcc  = 1e-5;end
if maxAngularAcc == 0, maxAngularAcc  = 1e-5;end
if maxLinearVel  == 0, maxLinearVel  = 1e-5;end
if maxAngularVel == 0, maxAngularVel = 1e-5;end

dxyz        = targetPose(1:3) - departPose(1:3);
dyaw        = targetPose(4) - departPose(4);
distance    = norm(dxyz);
twoMinDist  = maxLinearVel^2/maxLinearAcc;
distAngle   = abs(dyaw);
twoMinTheta = maxAngularVel^2/maxAngularAcc;

vel = zeros(4,1);
if distance > twoMinDist
    ta  = maxLinearVel/maxLinearAcc;
    tad = (distance - twoMinDist)/maxLinearVel;
    td  = ta + tad;
    te  = ta + td;
    if (t-departTime) < ta
        velxyz = maxLinearAcc*(t-departTime);
    elseif ta <= (t-departTime) && (t-departTime) < td
        velxyz = maxLinearVel;
    elseif td <= (t-departTime) && (t-departTime) < te
        velxyz = -maxLinearAcc*(t-departTime-td) + maxLinearVel;
    else
        velxyz = 0;
    end
else
    tp = sqrt(distance/maxLinearAcc);
    te = 2*tp;
    velp = maxLinearAcc*tp;
    if (t-departTime) < tp
        velxyz = maxLinearAcc*(t-departTime);
    elseif tp <= (t-departTime) && (t-departTime) < te
        velxyz = -maxLinearAcc*(t-departTime-tp)+velp;
    else
        velxyz = 0;
    end
end
if distance ~=0
    vel(1:3) = velxyz*dxyz/distance;
end

if distAngle > twoMinTheta
    ta  = maxAngularVel/maxAngularAcc;                   % acceleration period
    tad = (distAngle-twoMinTheta)/maxAngularVel; % acc to deceleration period
    td  = ta + tad;                  % start deceleration
    te  = ta + td;                   % end deceleration
    if (t-departTime) < ta
        omega = maxAngularAcc*(t-departTime);
    elseif ta <= (t-departTime) && (t-departTime) < td
        omega = maxAngularVel;
    elseif td <= (t-departTime) && (t-departTime) < te
        omega = -maxAngularAcc*(t-departTime-td) + maxAngularVel;
    else
        omega = 0;
    end
else
    tp = sqrt(distAngle/maxAngularAcc);
    te = 2*tp;
    omegap = maxAngularAcc*tp;
    if (t-departTime) < tp
        omega = maxAngularAcc*(t-departTime);
    elseif tp <= (t-departTime) && (t-departTime) <= te
        omega = -maxAngularAcc*(t-departTime-tp)+omegap;
    else
        omega = 0;
    end
end
vel(4) = omega*sign(dyaw);
if abs(Ts)<1e-6
    genAcc = [0;0;0;0];
else
    genAcc = (vel - prevVel)/Ts;
end
prevVel = vel;
%genAcc_row = genAcc';

== matlab function Forward_and_inverse_Both/Subsystem13/Define Relative angle1 ==
  settings: updateMethod=DISCRETE
  data: initialPose input; reset_angle input; rawangle input; angle output; status input
function angle = fcn(initialPose, reset_angle, rawangle, status)

% continuousangle is absolute angle
% angle is relative angle

persistent prevPsi2pi jump rawangle_0 set_angle
if isempty(prevPsi2pi)
    prevPsi2pi = 0; jump = 0; rawangle_0 = rawangle; set_angle = 0;
end

if abs(rawangle-prevPsi2pi) >  pi
    if rawangle > 0
        jump = jump - 1;
    else
        jump = jump + 1;
    end
end
prevPsi2pi = rawangle;

continuousangle = rawangle + jump*2*pi; % continuous value

if (status && ~set_angle), rawangle_0 = continuousangle; set_angle  = 1; end

if reset_angle, rawangle_0 = continuousangle; end

angle = continuousangle - rawangle_0 + initialPose;

== matlab function Forward_and_inverse_Both/Forward_Kinematic_Good1 ==
  data: Px output; Py output; Pz output; th1 input; th2 input; th3 input; th4 input; th5 input; th6 input
function [Px,Py,Pz] = forward_kinematics(th1, th2, th3, th4, th5, th6)
%All length in mm
l1=276;
l2=306;
a=79.75;
l3=160;
l4=227;
l5=70;
l6=38;
    % Compute DH transformation matrices
    A0 = dh_matrix(0    , 0     ,l1 , th1);   
    A1 = dh_matrix(0    ,-pi/2  ,0  , th2-pi/2);
    A2 = dh_matrix(l2   ,0      ,0  ,th3);
%     A3p= dh_matrix(a   ,0      ,0, 0);
    A3 = dh_matrix(a    ,-pi/2  ,0  ,th4);
    A4 = dh_matrix(0    ,0      ,l3+l4 ,0);
    A4p= dh_matrix(0   ,pi/2   ,0  ,th5);
    A5 = dh_matrix(0    ,-pi/2  , 0 ,th6);
    A6 = dh_matrix(0    ,0      ,l5+l6 ,0);
    
    % Total forward matrix H
    A0_6 = ( A0*A1 * A2 * A3 * A4 * A4p * A5 * A6) ;
    Px=A0_6(1,4);
    Py=A0_6(2,4);
    Pz=A0_6(3,4);

end
function A = dh_matrix(a , alpha ,d ,theta)
    A = [cos(theta)            , -sin(theta),           0       ,   a;
         cos(alpha)*sin(theta), cos(theta)*cos(alpha), -sin(alpha), -d*sin(alpha);
         sin(alpha)*sin(theta), sin(alpha)*cos(theta), cos(alpha), d*cos(alpha);
         0, 0, 0, 1];
end

== matlab function Forward_and_inverse_Both/Set Joint position to where it were left off/Joint4 ==
  data: pos input; posfinal output; pos_prev input; delta input
function posfinal = fcn(pos,pos_prev,delta)

if pos > 0        %%In case of clockwise rotation
    posc = pos_prev + abs(delta);
elseif pos < 0    %%In case of counter clockwise rotation
    posc = pos_prev - abs(delta);
else               %%Stay still if there's no input
    posc = pos_prev;
end

if posc <= 1 && posc >= -1.2 %%The joint only update its position if it stays within this range
    posfinal = posc;
else
    posfinal = pos_prev;
end

== matlab function Forward_and_inverse_Both/Set Joint position to where it were left off/MATLAB Function3 ==
  data: delta input; n input; y output; pos input; pos_prev input
function y = fcn(delta,n,pos,pos_prev)
if n == 0 && pos > 0
    pos = max(0,pos_prev - abs(delta));
elseif n == 0 && pos < 0
    pos = min(0,pos_prev + abs(delta));
end
y = pos;

== matlab function Forward_and_inverse_Both/Subsystem/MATLAB Function ==
  data: delta input; n input; y output; pos input; pos_prev input
function y = fcn(delta,n,pos,pos_prev)
if n == 0 && pos > 0
    pos = max(0,pos_prev - abs(delta));
elseif n == 0 && pos < 0
    pos = min(0,pos_prev + abs(delta));
end
y = pos;

== matlab function Forward_and_inverse_Both/Subsystem/MATLAB Function1 ==
  data: delta input; n input; y output; pos input; pos_prev input
function y = fcn(delta,n,pos,pos_prev)
if n == 0 && pos > 0
    pos = max(0,pos_prev - abs(delta));
elseif n == 0 && pos < 0
    pos = min(0,pos_prev + abs(delta));
end
y = pos;

== matlab function Forward_and_inverse_Both/Forward_Kinematic_Good5 ==
  data: Px output; Py output; Pz output; th1 input; th2 input; th3 input; th4 input; th5 input; th6 input
function [Px,Py,Pz] = forward_kinematics(th1, th2, th3, th4, th5, th6)
%All length in mm
l1=276;
l2=306;
a=79.75;
l3=160;
l4=227;
l5=70;
l6=38;
    % Compute DH transformation matrices
    A0 = dh_matrix(0    , 0     ,l1 , th1);   
    A1 = dh_matrix(0    ,-pi/2  ,0  , th2-pi/2);
    A2 = dh_matrix(l2   ,0      ,0  ,th3);
    A3p= dh_matrix(a   ,0      ,0, 0);
    A3 = dh_matrix(a    ,-pi/2  ,0  ,th4);
    A4 = dh_matrix(0    ,0      ,l3+l4 ,0);
    A4p= dh_matrix(0   ,pi/2   ,0  ,th5);
    A5 = dh_matrix(0    ,-pi/2  , 0 ,th6);
    A6 = dh_matrix(0    ,0      ,l5+l6 ,0);
    
    % Total forward matrix H
    A0_6 = ( A0*A1 * A2 * A3 * A4 * A4p * A5 * A6) ;
    Px=A0_6(1,4);
    Py=A0_6(2,4);
    Pz=A0_6(3,4);

end
function A = dh_matrix(a , alpha ,d ,theta)
    A = [cos(theta)            , -sin(theta),           0       ,   a;
         cos(alpha)*sin(theta), cos(theta)*cos(alpha), -sin(alpha), -d*sin(alpha);
         sin(alpha)*sin(theta), sin(alpha)*cos(theta), cos(alpha), d*cos(alpha);
         0, 0, 0, 1];
end

== matlab function Forward_and_inverse_Both/Inverse Kinematic ==
  settings: updateMethod=DISCRETE
  data: Px input; q1 output; Py input; Pz input; q2 output; q3 output; q4 output; q5 output; q6 output; R06 input
function [q1, q2, q3, q4, q5, q6] = inverseKinematics(Px, Py, Pz, R06)
    % Define actual geometry parameters (in mm)
    l1=276;
    l2=306;
    a=79.75;
    l3=160;
    l4=227;
    l5=70;
    l6=38;
    % Wrist position calculation
    O6=[Px,Py,Pz]';
    d6=l5+l6;
    OW = O6 - R06*[0;0;d6];
    % Compute wrist position (compensating for the end-effector offset)
    Pwx=OW(1);
    Pwy=OW(2);
    Pwz=OW(3);
    % Compute q1 directly from the wrist position
    q1 = atan2(Pwy, Pwx);
    r = sqrt(Pwx^2 + Pwy^2);
    h= Pwz-l1;
    % Intermediate calculations for q2 and q3
    s = sqrt(h^2 + r^2);
    alp = atan(h/r );
    w3 = l3 + l4;
    k3 = sqrt(a^2 + w3^2);
    beta = acos((l2^2 + s^2 - k3^2) / (2 * l2 * s));
    gamma = acos(( l2^2+k3^2-s^2) / (2 * l2 * k3));
    Phi = atan(w3/a);
    % Target angles for q2 and q3
    q2 = (-alp -beta+pi/2);
    q3 = (pi-gamma - Phi);

    % Compute R0_3 from q1, q2, q3
    R03 = [cos(q1)*cos(q2 + q3), -cos(q1)*sin(q2 + q3), -sin(q1);
           sin(q1)*cos(q2 + q3), -sin(q1)*sin(q2 + q3),  cos(q1);
           -sin(q2 + q3)       , -cos(q2 + q3)        , 0 ];
    R03t=transpose(R03);

    % Compute R3_6 from the known R0_3 and R0_6
    R3_6 = R03t* R06;

    % Extract elements from R3_6 for calculating q4, q5, q6
    s5c4 = -R3_6(1, 3);
    c5   = R3_6(2, 3);
    s5s4 = R3_6(3, 3);
    s5c6 = R3_6(2, 1);
    s5s6 = -R3_6(2, 2);

    % Joint angle q5

      q5p = atan2(-sqrt(1-c5^2),c5);
 % Joint angles q4 and q6
      q5=q5p;
        q4 = atan2(-s5s4, -s5c4);
        q6 = atan2(-s5s6, -s5c6);

end

== matlab function Forward_and_inverse_Both/Subsystem14/Define Relative angle1 ==
  settings: updateMethod=DISCRETE
  data: initialPose input; reset_angle input; rawangle input; angle output; status input
function angle = fcn(initialPose, reset_angle, rawangle, status)

% continuousangle is absolute angle
% angle is relative angle

persistent prevPsi2pi jump rawangle_0 set_angle
if isempty(prevPsi2pi)
    prevPsi2pi = 0; jump = 0; rawangle_0 = rawangle; set_angle = 0;
end

if abs(rawangle-prevPsi2pi) >  pi
    if rawangle > 0
        jump = jump - 1;
    else
        jump = jump + 1;
    end
end
prevPsi2pi = rawangle;

continuousangle = rawangle + jump*2*pi; % continuous value

if (status && ~set_angle), rawangle_0 = continuousangle; set_angle  = 1; end

if reset_angle, rawangle_0 = continuousangle; end

angle = continuousangle - rawangle_0 + initialPose;

== matlab function Forward_and_inverse_Both/Subsystem18/Define Relative angle1 ==
  settings: updateMethod=DISCRETE
  data: initialPose input; reset_angle input; rawangle input; angle output; status input
function angle = fcn(initialPose, reset_angle, rawangle, status)

% continuousangle is absolute angle
% angle is relative angle

persistent prevPsi2pi jump rawangle_0 set_angle
if isempty(prevPsi2pi)
    prevPsi2pi = 0; jump = 0; rawangle_0 = rawangle; set_angle = 0;
end

if abs(rawangle-prevPsi2pi) >  pi
    if rawangle > 0
        jump = jump - 1;
    else
        jump = jump + 1;
    end
end
prevPsi2pi = rawangle;

continuousangle = rawangle + jump*2*pi; % continuous value

if (status && ~set_angle), rawangle_0 = continuousangle; set_angle  = 1; end

if reset_angle, rawangle_0 = continuousangle; end

angle = continuousangle - rawangle_0 + initialPose;

== matlab function Forward_and_inverse_Both/Subsystem24/Define Relative angle1 ==
  settings: updateMethod=DISCRETE
  data: initialPose input; reset_angle input; rawangle input; angle output; status input
function angle = fcn(initialPose, reset_angle, rawangle, status)

% continuousangle is absolute angle
% angle is relative angle

persistent prevPsi2pi jump rawangle_0 set_angle
if isempty(prevPsi2pi)
    prevPsi2pi = 0; jump = 0; rawangle_0 = rawangle; set_angle = 0;
end

if abs(rawangle-prevPsi2pi) >  pi
    if rawangle > 0
        jump = jump - 1;
    else
        jump = jump + 1;
    end
end
prevPsi2pi = rawangle;

continuousangle = rawangle + jump*2*pi; % continuous value

if (status && ~set_angle), rawangle_0 = continuousangle; set_angle  = 1; end

if reset_angle, rawangle_0 = continuousangle; end

angle = continuousangle - rawangle_0 + initialPose;

== matlab function Forward_and_inverse_Both/Subsystem25/Define Relative angle ==
  settings: updateMethod=DISCRETE
  data: initialPose input; reset_angle input; rawangle input; angle output; status input
function angle = fcn(initialPose, reset_angle, rawangle, status)

% continuousangle is absolute angle
% angle is relative angle

persistent prevPsi2pi jump rawangle_0 set_angle
if isempty(prevPsi2pi)
    prevPsi2pi = 0; jump = 0; rawangle_0 = rawangle; set_angle = 0;
end

if abs(rawangle-prevPsi2pi) >  pi
    if rawangle > 0
        jump = jump - 1;
    else
        jump = jump + 1;
    end
end
if abs(rawangle-prevPsi2pi) >  pi/2 && abs(rawangle-prevPsi2pi) < pi
    if rawangle > 0
        jump = jump - 1/2;
    else
        jump = jump + 1/2;
    end
end

prevPsi2pi = rawangle;

continuousangle = rawangle + jump*2*pi; % continuous value

if (status && ~set_angle), rawangle_0 = continuousangle; set_angle  = 1; end

if reset_angle, rawangle_0 = continuousangle; end

angle = continuousangle - rawangle_0 + initialPose;

== matlab function Forward_and_inverse_Both/Inverse Kinematic4 ==
  settings: updateMethod=DISCRETE
  data: Px input; q1 output; Py input; Pz input; q2 output; q3 output; q4 output; q5 output; q6 output; R06 input
function [q1, q2, q3, q4, q5, q6] = inverseKinematics(Px, Py, Pz, R06)
    % Define actual geometry parameters (in mm)
    l1 = 276;
    l2 = 306;
    a = 79.75;
    l3 = 160;
    l4 = 227;
    l5 = 70;
    l6 = 38;

    % Wrist position calculation
    O6 = [Px, Py, Pz]';
    d6 = l5 + l6;
    OW = O6 - R06 * [0; 0; d6];

    % Compute wrist position (compensating for the end-effector offset)
    Pwx = OW(1);
    Pwy = OW(2);
    Pwz = OW(3);

    % Compute q1 directly from the wrist position
    q1 = atan2(Pwy, Pwx);
    r = sqrt(Pwx^2 + Pwy^2);
    h = Pwz - l1;

    % Intermediate calculations for q2 and q3
    s = sqrt(h^2 + r^2);
    alp = atan(h / r);
    w3 = l3 + l4;
    k3 = sqrt(a^2 + w3^2);

    % Clamp inputs for acos to avoid complex results
    beta_input = (l2^2 + s^2 - k3^2) / (2 * l2 * s);
    beta_input = max(-1, min(1, beta_input)); % Clamp to [-1, 1]
    beta = acos(beta_input);

    gamma_input = (l2^2 + k3^2 - s^2) / (2 * l2 * k3);
    gamma_input = max(-1, min(1, gamma_input)); % Clamp to [-1, 1]
    gamma = acos(gamma_input);

    Phi = atan(w3 / a);

    % Target angles for q2 and q3
    q2 = (-alp - beta + pi / 2);
    q3 = (pi - gamma - Phi);

    % Compute R0_3 from q1, q2, q3
    R03 = [cos(q1) * cos(q2 + q3), -cos(q1) * sin(q2 + q3), -sin(q1);
           sin(q1) * cos(q2 + q3), -sin(q1) * sin(q2 + q3),  cos(q1);
           -sin(q2 + q3),           -cos(q2 + q3),           0];
    R03t = transpose(R03);

    % Compute R3_6 from the known R0_3 and R0_6
    R3_6 = R03t * R06;

    % Extract elements from R3_6 for calculating q4, q5, q6
    s5c4 = -R3_6(1, 3);
    c5 = R3_6(2, 3);
    s5s4 = R3_6(3, 3);
    s5c6 = R3_6(2, 1);
    s5s6 = -R3_6(2, 2);

    % Joint angle q5
    q5 = atan2(-sqrt(max(0, 1 - c5^2)), c5); % Ensure non-negative argument for sqrt

    % Joint angles q4 and q6
    if abs(q5) > 1e-6
        q4 = atan2(-s5s4, -s5c4);
        q6 = atan2(-s5s6, -s5c6);
    else
        q4 = 0;
        q6 = atan2(R3_6(1, 2), R3_6(1, 1));
    end
end
